simulink model "UAV_Z_PID"  (R2020a)
settings: Solver=VariableStepAuto  StartTime=0.0  StopTime=inf  RelTol=1e-3
libraries: simulink x4, sharedtransform x1, robotuavlib x1
settings Model: Creator=chand  LastModifiedBy=nishi
settings SolverCC: AlgebraicLoopSolver=LineSearch

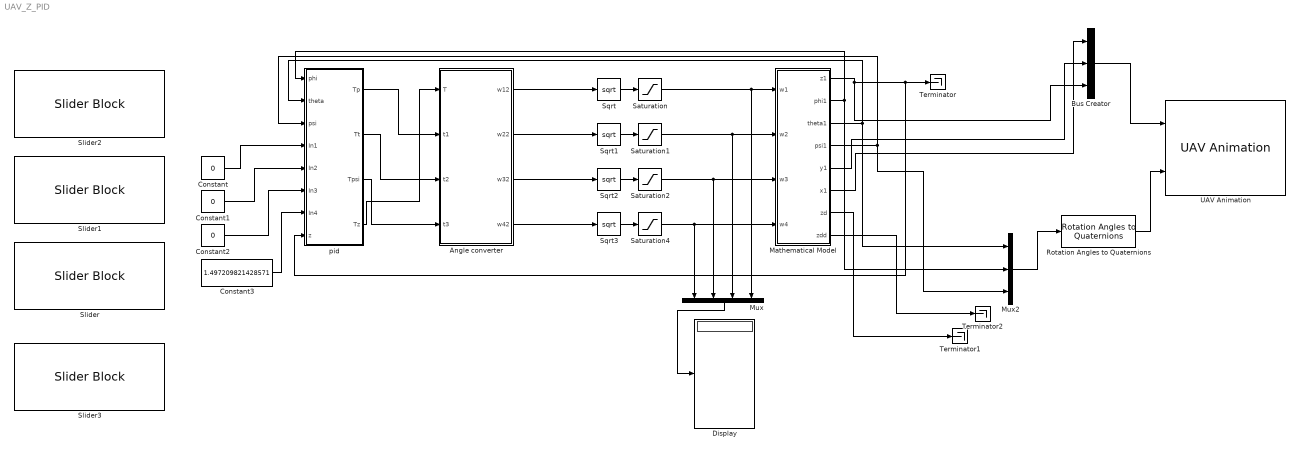
== system UAV_Z_PID ==
  Angle converter : MATLAB Function  TreatAsAtomicUnit=on
  Bus Creator : BusCreator  Inputs=3
  Constant : Constant  Value=0
  Constant1 : Constant  Value=0
  Constant2 : Constant  Value=0
  Constant3 : Constant  Value=1.497209821428571
  Display : Display
  Mathematical Model : Subsystem
  Mux : Mux
  Mux2 : Mux  Inputs=3
  Rotation Angles to Quaternions : sharedtransform/Rotation Angles to Quaternions  rotationOrder=XYZ  aMode=aMode
      settings: SourceProductBaseCode=AE,PW,MT,VE,VP
  Saturation{,1..2,4} (4 alike) : Saturate  UpperLimit=8000  LowerLimit=0
  Slider : SliderBlock  ScaleMin=-0.5236  ScaleMax=0.5236
  Slider1 : SliderBlock  ScaleMin=-0.5236  ScaleMax=0.5236
  Slider2 : SliderBlock  ScaleMin=-0.5236  ScaleMax=0.5236
  Slider3 : SliderBlock  ScaleMin=1  ScaleMax=10
  Sqrt{,1..3} (4 alike) : Sqrt  SaturateOnIntegerOverflow=on
  Terminator : Terminator
  Terminator1 : Terminator
  Terminator2 : Terminator
  UAV Animation : robotuavlib/UAV Animation  UAVType=Multirotor  UAVSize=1  InertialZDirection=Up  SampleTime=-1
      settings: SourceProductBaseCode=ROBOTICS_UAV_LIB
  pid : Subsystem
  wires:
  Constant/1 -> pid/4(In1)
  Constant1/1 -> pid/5(In2)
  Constant2/1 -> pid/6(In3)
  Constant3/1 -> pid/7(In4)
  pid/1(Tp) -> Angle converter/2(t1)
  pid/2(Tt) -> Angle converter/3(t2)
  pid/3(Tpsi) -> Angle converter/4(t3)
  Sqrt/1 -> Saturation/1
  Sqrt1/1 -> Saturation1/1
  Sqrt3/1 -> Saturation4/1
  Sqrt2/1 -> Saturation2/1
  Mux/1 -> Display/1
  Angle converter/3(w32) -> Sqrt2/1
  Angle converter/4(w42) -> Sqrt3/1
  Angle converter/2(w22) -> Sqrt1/1
  Angle converter/1(w12) -> Sqrt/1
  Saturation4/1 -> Mux/1, Mathematical Model/4(w4)
  Saturation2/1 -> Mux/2, Mathematical Model/3(w3)
  Saturation1/1 -> Mux/3, Mathematical Model/2(w2)
  Saturation/1 -> Mux/4, Mathematical Model/1(w1)
  Mathematical Model/1(z1) -> Bus Creator/3, pid/8(z), Terminator/1
  Mathematical Model/2(phi1) -> Mux2/2, pid/1(phi)
  Mathematical Model/3(theta1) -> Mux2/1, pid/2(theta)
  Mathematical Model/4(psi1) -> Mux2/3, pid/3(psi)
  pid/4(Tz) -> Angle converter/1(T)
  Mathematical Model/6(x1) -> Bus Creator/1
  Mathematical Model/5(y1) -> Bus Creator/2
  Mux2/1 -> Rotation Angles to Quaternions/1
  Rotation Angles to Quaternions/1 -> UAV Animation/2
  Bus Creator/1 -> UAV Animation/1
  Mathematical Model/7(zd) -> Terminator1/1
  Mathematical Model/8(zdd) -> Terminator2/1

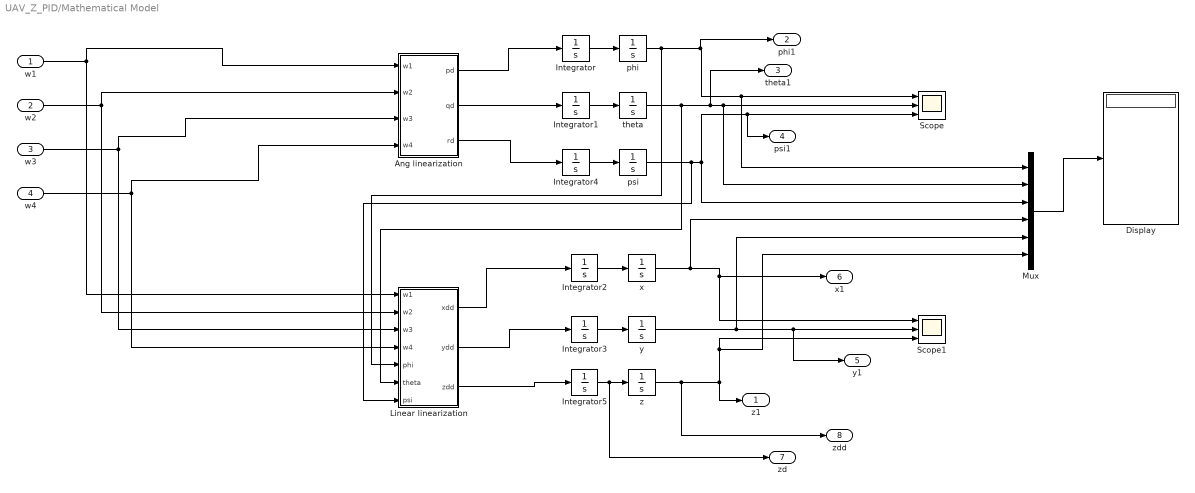
== system UAV_Z_PID/Mathematical Model ==
  w1 : Inport
  w2 : Inport  Port=2
  w3 : Inport  Port=3
  w4 : Inport  Port=4
  Ang linearization : MATLAB Function  TreatAsAtomicUnit=on
  Display : Display
  Integrator{,1..5} (6 alike) : Integrator
  Linear linearization : MATLAB Function  TreatAsAtomicUnit=on
  Mux : Mux  Inputs=6
  Scope : Scope  NumInputPorts=3
  Scope1 : Scope  NumInputPorts=3
  phi : Integrator
  psi : Integrator
  theta : Integrator
  x : Integrator
  y : Integrator
  z : Integrator
  z1 : Outport
  phi1 : Outport  Port=2
  theta1 : Outport  Port=3
  psi1 : Outport  Port=4
  y1 : Outport  Port=5
  x1 : Outport  Port=6
  zd : Outport  Port=7
  zdd : Outport  Port=8
  wires:
  w3/1 -> Ang linearization/3(w3), Linear linearization/3(w3)
  w4/1 -> Ang linearization/4(w4), Linear linearization/4(w4)
  w1/1 -> Ang linearization/1(w1), Linear linearization/1(w1)
  Integrator5/1 -> zd/1, z/1
  Ang linearization/2(qd) -> Integrator1/1
  psi/1 -> Linear linearization/7(psi), psi1/1, Scope/3, Mux/3
  Mux/1 -> Display/1
  Integrator4/1 -> psi/1
  w2/1 -> Ang linearization/2(w2), Linear linearization/2(w2)
  Ang linearization/3(rd) -> Integrator4/1
  Linear linearization/2(ydd) -> Integrator3/1
  theta/1 -> Linear linearization/6(theta), theta1/1, Mux/2, Scope/2
  Linear linearization/3(zdd) -> Integrator5/1
  phi/1 -> Linear linearization/5(phi), phi1/1, Mux/1, Scope/1
  Integrator2/1 -> x/1
  Integrator3/1 -> y/1
  Linear linearization/1(xdd) -> Integrator2/1
  Integrator1/1 -> theta/1
  x/1 -> Mux/4, Scope1/1, x1/1
  z/1 -> zdd/1, Mux/6, Scope1/3, z1/1
  Ang linearization/1(pd) -> Integrator/1
  Integrator/1 -> phi/1
  y/1 -> Mux/5, y1/1, Scope1/2

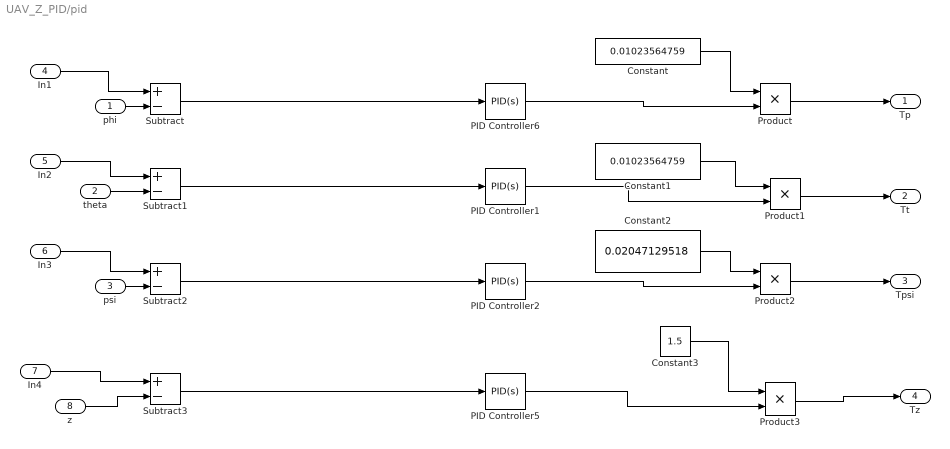
== system UAV_Z_PID/pid ==
  phi : Inport
  theta : Inport  Port=2
  psi : Inport  Port=3
  In1 : Inport  Port=4
  In2 : Inport  Port=5
  In3 : Inport  Port=6
  In4 : Inport  Port=7
  z : Inport  Port=8
  Constant : Constant  Value=0.01023564759
  Constant1 : Constant  Value=0.01023564759
  Constant2 : Constant  Value=0.02047129518
  Constant3 : Constant  Value=1.5
  PID Controller1 : simulink/Continuous/PID Controller  Controller=PID  Form=Parallel  TimeDomain=Continuous-time  UseExternalTs=off  SampleTime=-1  IntegratorMethod=Forward Euler  FilterMethod=Forward Euler  ControllerParametersSource=internal  P=48247.4967638302  I=18465.7739956786  D=30690.8552975803  UseFilter=on  N=1091.39224421761  TunerSelectOption=Transfer Function Based (PID Tuner App)  InitialConditionSource=internal  InitialConditionForIntegrator=0  InitialConditionForFilter=0  DifferentiatorICPrevScaledInput=0  ExternalReset=none  TrackingMode=off  Kt=1  LimitOutput=off  UpperSaturationLimit=inf  LowerSaturationLimit=-inf  LinearizeAsGain=on  AntiWindupMode=none  Kb=1  POutMin=[]  POutMax=[]  IOutMin=[]  IOutMax=[]  DOutMin=[]  DOutMax=[]  NOutMin=[]  NOutMax=[]  SumOutMin=[]  SumOutMax=[]  SaturationOutMin=[]  SaturationOutMax=[]  PParamMin=[]  PParamMax=[]  IParamMin=[]  IParamMax=[]  DParamMin=[]  DParamMax=[]  NParamMin=[]  NParamMax=[]  KbParamMin=[]  KbParamMax=[]  KtParamMin=[]  KtParamMax=[]  KbOutMin=[]  KbOutMax=[]  KtOutMin=[]  KtOutMax=[]  IntegratorOutMin=[]  IntegratorOutMax=[]  FilterOutMin=[]  FilterOutMax=[]  SumI1OutMin=[]  SumI1OutMax=[]  SumI2OutMin=[]  SumI2OutMax=[]  SumI3OutMin=[]  SumI3OutMax=[]  SumI4OutMin=[]  SumI4OutMax=[]  SumDOutMin=[]  SumDOutMax=[]  DifferentiatorOutMin=[]  DifferentiatorOutMax=[]  FilterDiffOutCoefMin=[]  FilterDiffOutCoefMax=[]  ReciprocalOutMin=[]  ReciprocalOutMax=[]  SumDenOutMin=[]  SumDenOutMax=[]  SumNumOutMin=[]  SumNumOutMax=[]  DivideOutMin=[]  DivideOutMax=[]  UdiffTsProdOutMin=[]  UdiffTsProdOutMax=[]  NTsProdOutMin=[]  NTsProdOutMax=[]  UintegralTsProdOutMin=[]  UintegralTsProdOutMax=[]  UngainTsProdOutMin=[]  UngainTsProdOutMax=[]  IntegratorContinuousStateAttributes=''  IntegratorStateMustResolveToSignalObject=off  IntegratorRTWStateStorageClass=Auto  FilterContinuousStateAttributes=''  FilterStateMustResolveToSignalObject=off  FilterRTWStateStorageClass=Auto  ParallelPVariant=InternalParameters  IdealPVariant=Disabled  IVariant=InternalParameters  DVariant=InternalParameters  IntegratorVariant=Continuous  SatVariant=Disabled  AWVariant=Passthrough  PCopyVariant=Disabled  TRVariant=Disabled  FdbkBlocksVariant=Forward  IdealPFdbkVariant=Disabled  SatFdbkVariant=Disabled  DerivativeFilterVariant=ContFilter  NVariant=InternalParameters  NCopyVariant=Disabled  FilterICVariant=InternalICsFilter  IntegratorICVariant=InternalICs  ExternalResetVariant=Disabled  TRSumVariant=Passthrough  SumFdbkVariant=Disabled  SumVariant=Sum_PID  TsampFilterVariant=InternalTs  TsampNgainVariant=Passthrough  TsampIntegralVariant=Passthrough
  PID Controller2 : simulink/Continuous/PID Controller  Controller=PID  Form=Parallel  TimeDomain=Continuous-time  UseExternalTs=off  SampleTime=-1  IntegratorMethod=Forward Euler  FilterMethod=Forward Euler  ControllerParametersSource=internal  P=39829.3758447558  I=12433.1764016541  D=29338.3718993805  UseFilter=on  N=1042.27150166912  TunerSelectOption=Transfer Function Based (PID Tuner App)  InitialConditionSource=internal  InitialConditionForIntegrator=0  InitialConditionForFilter=0  DifferentiatorICPrevScaledInput=0  ExternalReset=none  TrackingMode=off  Kt=1  LimitOutput=off  UpperSaturationLimit=inf  LowerSaturationLimit=-inf  LinearizeAsGain=on  AntiWindupMode=none  Kb=1  POutMin=[]  POutMax=[]  IOutMin=[]  IOutMax=[]  DOutMin=[]  DOutMax=[]  NOutMin=[]  NOutMax=[]  SumOutMin=[]  SumOutMax=[]  SaturationOutMin=[]  SaturationOutMax=[]  PParamMin=[]  PParamMax=[]  IParamMin=[]  IParamMax=[]  DParamMin=[]  DParamMax=[]  NParamMin=[]  NParamMax=[]  KbParamMin=[]  KbParamMax=[]  KtParamMin=[]  KtParamMax=[]  KbOutMin=[]  KbOutMax=[]  KtOutMin=[]  KtOutMax=[]  IntegratorOutMin=[]  IntegratorOutMax=[]  FilterOutMin=[]  FilterOutMax=[]  SumI1OutMin=[]  SumI1OutMax=[]  SumI2OutMin=[]  SumI2OutMax=[]  SumI3OutMin=[]  SumI3OutMax=[]  SumI4OutMin=[]  SumI4OutMax=[]  SumDOutMin=[]  SumDOutMax=[]  DifferentiatorOutMin=[]  DifferentiatorOutMax=[]  FilterDiffOutCoefMin=[]  FilterDiffOutCoefMax=[]  ReciprocalOutMin=[]  ReciprocalOutMax=[]  SumDenOutMin=[]  SumDenOutMax=[]  SumNumOutMin=[]  SumNumOutMax=[]  DivideOutMin=[]  DivideOutMax=[]  UdiffTsProdOutMin=[]  UdiffTsProdOutMax=[]  NTsProdOutMin=[]  NTsProdOutMax=[]  UintegralTsProdOutMin=[]  UintegralTsProdOutMax=[]  UngainTsProdOutMin=[]  UngainTsProdOutMax=[]  IntegratorContinuousStateAttributes=''  IntegratorStateMustResolveToSignalObject=off  IntegratorRTWStateStorageClass=Auto  FilterContinuousStateAttributes=''  FilterStateMustResolveToSignalObject=off  FilterRTWStateStorageClass=Auto  ParallelPVariant=InternalParameters  IdealPVariant=Disabled  IVariant=InternalParameters  DVariant=InternalParameters  IntegratorVariant=Continuous  SatVariant=Disabled  AWVariant=Passthrough  PCopyVariant=Disabled  TRVariant=Disabled  FdbkBlocksVariant=Forward  IdealPFdbkVariant=Disabled  SatFdbkVariant=Disabled  DerivativeFilterVariant=ContFilter  NVariant=InternalParameters  NCopyVariant=Disabled  FilterICVariant=InternalICsFilter  IntegratorICVariant=InternalICs  ExternalResetVariant=Disabled  TRSumVariant=Passthrough  SumFdbkVariant=Disabled  SumVariant=Sum_PID  TsampFilterVariant=InternalTs  TsampNgainVariant=Passthrough  TsampIntegralVariant=Passthrough
  PID Controller5 : simulink/Continuous/PID Controller  Controller=PID  Form=Parallel  TimeDomain=Continuous-time  UseExternalTs=off  SampleTime=-1  IntegratorMethod=Forward Euler  FilterMethod=Forward Euler  ControllerParametersSource=internal  P=22085.7324832454  I=6287.67958211652  D=17837.9242830577  UseFilter=on  N=950.562907073997  TunerSelectOption=Transfer Function Based (PID Tuner App)  InitialConditionSource=internal  InitialConditionForIntegrator=0  InitialConditionForFilter=0  DifferentiatorICPrevScaledInput=0  ExternalReset=none  TrackingMode=off  Kt=1  LimitOutput=off  UpperSaturationLimit=inf  LowerSaturationLimit=-inf  LinearizeAsGain=on  AntiWindupMode=none  Kb=1  POutMin=[]  POutMax=[]  IOutMin=[]  IOutMax=[]  DOutMin=[]  DOutMax=[]  NOutMin=[]  NOutMax=[]  SumOutMin=[]  SumOutMax=[]  SaturationOutMin=[]  SaturationOutMax=[]  PParamMin=[]  PParamMax=[]  IParamMin=[]  IParamMax=[]  DParamMin=[]  DParamMax=[]  NParamMin=[]  NParamMax=[]  KbParamMin=[]  KbParamMax=[]  KtParamMin=[]  KtParamMax=[]  KbOutMin=[]  KbOutMax=[]  KtOutMin=[]  KtOutMax=[]  IntegratorOutMin=[]  IntegratorOutMax=[]  FilterOutMin=[]  FilterOutMax=[]  SumI1OutMin=[]  SumI1OutMax=[]  SumI2OutMin=[]  SumI2OutMax=[]  SumI3OutMin=[]  SumI3OutMax=[]  SumI4OutMin=[]  SumI4OutMax=[]  SumDOutMin=[]  SumDOutMax=[]  DifferentiatorOutMin=[]  DifferentiatorOutMax=[]  FilterDiffOutCoefMin=[]  FilterDiffOutCoefMax=[]  ReciprocalOutMin=[]  ReciprocalOutMax=[]  SumDenOutMin=[]  SumDenOutMax=[]  SumNumOutMin=[]  SumNumOutMax=[]  DivideOutMin=[]  DivideOutMax=[]  UdiffTsProdOutMin=[]  UdiffTsProdOutMax=[]  NTsProdOutMin=[]  NTsProdOutMax=[]  UintegralTsProdOutMin=[]  UintegralTsProdOutMax=[]  UngainTsProdOutMin=[]  UngainTsProdOutMax=[]  IntegratorContinuousStateAttributes=''  IntegratorStateMustResolveToSignalObject=off  IntegratorRTWStateStorageClass=Auto  FilterContinuousStateAttributes=''  FilterStateMustResolveToSignalObject=off  FilterRTWStateStorageClass=Auto  ParallelPVariant=InternalParameters  IdealPVariant=Disabled  IVariant=InternalParameters  DVariant=InternalParameters  IntegratorVariant=Continuous  SatVariant=Disabled  AWVariant=Passthrough  PCopyVariant=Disabled  TRVariant=Disabled  FdbkBlocksVariant=Forward  IdealPFdbkVariant=Disabled  SatFdbkVariant=Disabled  DerivativeFilterVariant=ContFilter  NVariant=InternalParameters  NCopyVariant=Disabled  FilterICVariant=InternalICsFilter  IntegratorICVariant=InternalICs  ExternalResetVariant=Disabled  TRSumVariant=Passthrough  SumFdbkVariant=Disabled  SumVariant=Sum_PID  TsampFilterVariant=InternalTs  TsampNgainVariant=Passthrough  TsampIntegralVariant=Passthrough
  PID Controller6 : simulink/Continuous/PID Controller  Controller=PID  Form=Parallel  TimeDomain=Continuous-time  UseExternalTs=off  SampleTime=-1  IntegratorMethod=Forward Euler  FilterMethod=Forward Euler  ControllerParametersSource=internal  P=27671.2543764538  I=2174.07739566126  D=32285.7286533013  UseFilter=on  N=1142.8279760416  TunerSelectOption=Transfer Function Based (PID Tuner App)  InitialConditionSource=internal  InitialConditionForIntegrator=0  InitialConditionForFilter=0  DifferentiatorICPrevScaledInput=0  ExternalReset=none  TrackingMode=off  Kt=1  LimitOutput=off  UpperSaturationLimit=inf  LowerSaturationLimit=-inf  LinearizeAsGain=on  AntiWindupMode=none  Kb=1  POutMin=[]  POutMax=[]  IOutMin=[]  IOutMax=[]  DOutMin=[]  DOutMax=[]  NOutMin=[]  NOutMax=[]  SumOutMin=[]  SumOutMax=[]  SaturationOutMin=[]  SaturationOutMax=[]  PParamMin=[]  PParamMax=[]  IParamMin=[]  IParamMax=[]  DParamMin=[]  DParamMax=[]  NParamMin=[]  NParamMax=[]  KbParamMin=[]  KbParamMax=[]  KtParamMin=[]  KtParamMax=[]  KbOutMin=[]  KbOutMax=[]  KtOutMin=[]  KtOutMax=[]  IntegratorOutMin=[]  IntegratorOutMax=[]  FilterOutMin=[]  FilterOutMax=[]  SumI1OutMin=[]  SumI1OutMax=[]  SumI2OutMin=[]  SumI2OutMax=[]  SumI3OutMin=[]  SumI3OutMax=[]  SumI4OutMin=[]  SumI4OutMax=[]  SumDOutMin=[]  SumDOutMax=[]  DifferentiatorOutMin=[]  DifferentiatorOutMax=[]  FilterDiffOutCoefMin=[]  FilterDiffOutCoefMax=[]  ReciprocalOutMin=[]  ReciprocalOutMax=[]  SumDenOutMin=[]  SumDenOutMax=[]  SumNumOutMin=[]  SumNumOutMax=[]  DivideOutMin=[]  DivideOutMax=[]  UdiffTsProdOutMin=[]  UdiffTsProdOutMax=[]  NTsProdOutMin=[]  NTsProdOutMax=[]  UintegralTsProdOutMin=[]  UintegralTsProdOutMax=[]  UngainTsProdOutMin=[]  UngainTsProdOutMax=[]  IntegratorContinuousStateAttributes=''  IntegratorStateMustResolveToSignalObject=off  IntegratorRTWStateStorageClass=Auto  FilterContinuousStateAttributes=''  FilterStateMustResolveToSignalObject=off  FilterRTWStateStorageClass=Auto  ParallelPVariant=InternalParameters  IdealPVariant=Disabled  IVariant=InternalParameters  DVariant=InternalParameters  IntegratorVariant=Continuous  SatVariant=Disabled  AWVariant=Passthrough  PCopyVariant=Disabled  TRVariant=Disabled  FdbkBlocksVariant=Forward  IdealPFdbkVariant=Disabled  SatFdbkVariant=Disabled  DerivativeFilterVariant=ContFilter  NVariant=InternalParameters  NCopyVariant=Disabled  FilterICVariant=InternalICsFilter  IntegratorICVariant=InternalICs  ExternalResetVariant=Disabled  TRSumVariant=Passthrough  SumFdbkVariant=Disabled  SumVariant=Sum_PID  TsampFilterVariant=InternalTs  TsampNgainVariant=Passthrough  TsampIntegralVariant=Passthrough
  Product{,1..3} (4 alike) : Product
  Subtract{,1..3} (4 alike) : Sum  Inputs=+-
  Tp : Outport
  Tt : Outport  Port=2
  Tpsi : Outport  Port=3
  Tz : Outport  Port=4
  wires:
  phi/1 -> Subtract/2
  Subtract/1 -> PID Controller6/1
  Subtract1/1 -> PID Controller1/1
  Subtract2/1 -> PID Controller2/1
  theta/1 -> Subtract1/2
  psi/1 -> Subtract2/2
  In1/1 -> Subtract/1
  In2/1 -> Subtract1/1
  In3/1 -> Subtract2/1
  Product2/1 -> Tpsi/1
  Product1/1 -> Tt/1
  Product/1 -> Tp/1
  Constant/1 -> Product/1
  Constant2/1 -> Product2/1
  Constant1/1 -> Product1/1
  PID Controller6/1 -> Product/2
  PID Controller1/1 -> Product1/2
  PID Controller2/1 -> Product2/2
  Constant3/1 -> Product3/1
  Product3/1 -> Tz/1
  PID Controller5/1 -> Product3/2
  Subtract3/1 -> PID Controller5/1
  In4/1 -> Subtract3/1
  z/1 -> Subtract3/2

== matlab function UAV_Z_PID/Mathematical Model/Linear linearization ==
  data: w1 input; xdd output; w2 input; w3 input; w4 input; phi input; theta input; psi input; ydd output; zdd output
function [xdd,ydd,zdd] = fcn(w1,w2,w3,w4,phi,theta,psi)
g=9.81;
m=1.5;
ct=8.586e-08;
tt=ct*(w1^2 + w2^2 + w3^2 + w4^2);
xdd=(phi*(sin(psi))  + theta*(cos(psi)))*tt/m;
ydd=(theta*(sin(phi)) - phi*(cos(psi)))*tt/m;
% zdd=-m*g+tt;
if tt<=m*g
    zdd=0;
else
    zdd=-m*g+tt;
end

== matlab function UAV_Z_PID/Mathematical Model/Ang linearization ==
  data: w1 input; pd output; w2 input; w3 input; w4 input; qd output; rd output
function [pd,qd,rd] = fcn(w1,w2,w3,w4)
d=0.176777;ct=8.586e-08;cq=4.81e-09;
Jxx=0.01023564759;Jyy=0.01023564759;Jzz=0.02047129518;
pd=(d*ct*(-w1^2 + w2^2 + w3^2 - w4^2)/(Jxx*1.414));
qd=(d*ct*(-w1^2 - w2^2 + w3^2 + w4^2)/(Jyy*1.414));
rd=(cq*(-w1^2 + w2^2 - w3^2 + w4^2)/Jzz);

== matlab function UAV_Z_PID/Angle converter ==
  data: T input; w12 output; t1 input; t2 input; t3 input; w22 output; w32 output; w42 output
function [w12,w22,w32,w42]  = fcn(T,t1,t2,t3)
d=0.176777;ct=8.586e-08;cq=4.81e-09;
A=[ct ct ct ct; -(d*ct) (d*ct) (d*ct) -(d*ct); -d*ct -d*ct d*ct d*ct;-cq cq -cq cq];
B=[T t1*1.414 t2*1.414 t3]';
C=inv(A)*B;
w12=C(1,1);
w22=C(2,1);w32=C(3,1);w42=C(4,1);
if(w12<0)
    w12=0;
end
if(w22<0)
    w22=0;
end
if(w32<0)
    w32=0;
end
if(w42<0)
    w42=0;
end
% T=ct*(a + b + c + e);
% t1=d*ct*(-a + b + c - e)/1.414;
% t2=d*ct*(-a - b + c + e)/1.414;
% t3=cq*d*(-a + b - c + e);
% sol=solve(T,t1,t2,t3);
% w2=T+t3+t2+t1;
% w1=T-t3+t2-t1;
% w3=T+t3-t2-t1;
% w4=T-t3-t2+t1;
